simulink model "modelP16"  (R2014b)
settings: Solver=ode4  StartTime=0.0  StopTime=TIME_SIM  FixedStep=STEP_SIZE  RelTol=1e-3
values from neighbouring files (symbols this model uses):
  Bd = [B B]    [mainbis.m]
  C = [1 0 0]    [mainbis.m]
  K = acker(F,G,Pdisc)    [mainbis.m]
  N = inv(C*inv(eye(3)-Fk)*G)    [mainbis.m]
  Ts = 0.0002    [mainbis.m]
undefined symbols (not defined in the file or in its folder): A, B
settings Model: Creator=Kate  LastModifiedBy=Kate
settings DataIOCC: SaveState=on
settings DebuggingCC: MultiTaskRateTransMsg=warning

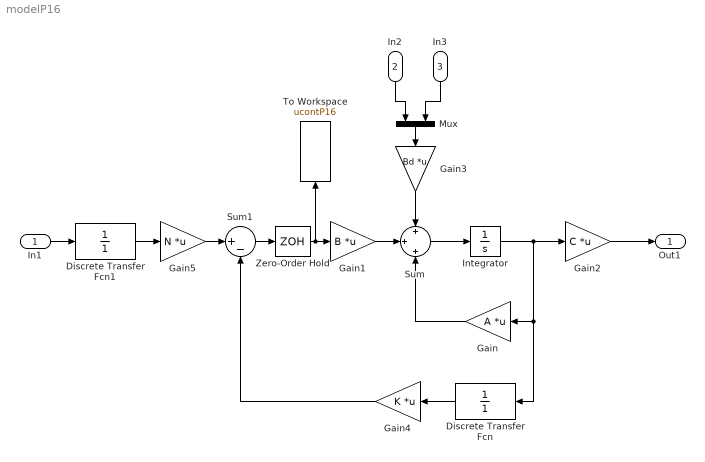
== system modelP16 ==
  In1 : Inport
  In2 : Inport  Port=2
  In3 : Inport  Port=3
  Discrete Transfer Fcn : DiscreteTransferFcn  Denominator=[1]  SampleTime=Ts
  Discrete Transfer Fcn1 : DiscreteTransferFcn  Denominator=[1]  SampleTime=Ts
  Gain : Gain  Gain=A  Multiplication=Matrix(K*u)
  Gain1 : Gain  Gain=B  Multiplication=Matrix(K*u)
  Gain2 : Gain  Gain=C  Multiplication=Matrix(K*u)
  Gain3 : Gain  Gain=Bd  Multiplication=Matrix(K*u)
  Gain4 : Gain  Gain=K  Multiplication=Matrix(K*u)  SampleTime=Ts
  Gain5 : Gain  Gain=N  Multiplication=Matrix(K*u)  SampleTime=Ts
  Integrator : Integrator
  Mux : Mux  Inputs=2
  Sum : Sum  Inputs=+|+|+
  Sum1 : Sum  Inputs=|+-
  To Workspace : ToWorkspace  VariableName=ucontP16  SaveFormat=Timeseries  SampleTime=-1
  Zero-Order Hold : ZeroOrderHold  SampleTime=Ts
  Out1 : Outport
  wires:
  Sum/1 -> Integrator/1
  Integrator/1 -> Gain2/1, Discrete Transfer Fcn/1, Gain/1
  Gain/1 -> Sum/3
  Gain1/1 -> Sum/2
  Gain2/1 -> Out1/1
  Gain3/1 -> Sum/1
  Mux/1 -> Gain3/1
  In2/1 -> Mux/1
  In3/1 -> Mux/2
  Gain5/1 -> Sum1/1
  Gain4/1 -> Sum1/2
  Discrete Transfer Fcn/1 -> Gain4/1
  Sum1/1 -> Zero-Order Hold/1
  Zero-Order Hold/1 -> To Workspace/1, Gain1/1
  Discrete Transfer Fcn1/1 -> Gain5/1
  In1/1 -> Discrete Transfer Fcn1/1
